simulink model "rl_17b"  (R2017b)
settings: Solver=VariableStepAuto  StartTime=0.0  StopTime=0.08  MaxStep=1e-4  RelTol=1e-8
values from neighbouring files (symbols this model uses):
  F_b = 50.0    (= 50)    [rl2_ini.m]    (also in rl_ini.m; rl_ini_jm.m; rlc_gformer_ini.m)
  L = 1e-3    (= 0.001)    [rl_ini.m]    (also in rl_ini_jm.m)
  Lmat = Lmat_km*Lenght    [rl_ini_jm.m]
  params_pu = [S_b,U_b,Omega_b,R,L]    [rl_ini.m]    (also in rl_ini_jm.m)
  R = 1.0    (= 1)    [rl_ini.m]    (also in rl_ini_jm.m)
  Rmat = Rmat_km*Lenght    [rl_ini_jm.m]
undefined symbols (not defined in the file or in its folder): T_s_power
libraries: powerlib x19, powerlib_meascontrol x8
settings Model: Creator=jmmauricio  LastModifiedBy=jmmau
settings CodeAppCC: StateflowObjectComments=on
settings SimscapeCC: SimscapeNormalizeSystem=off

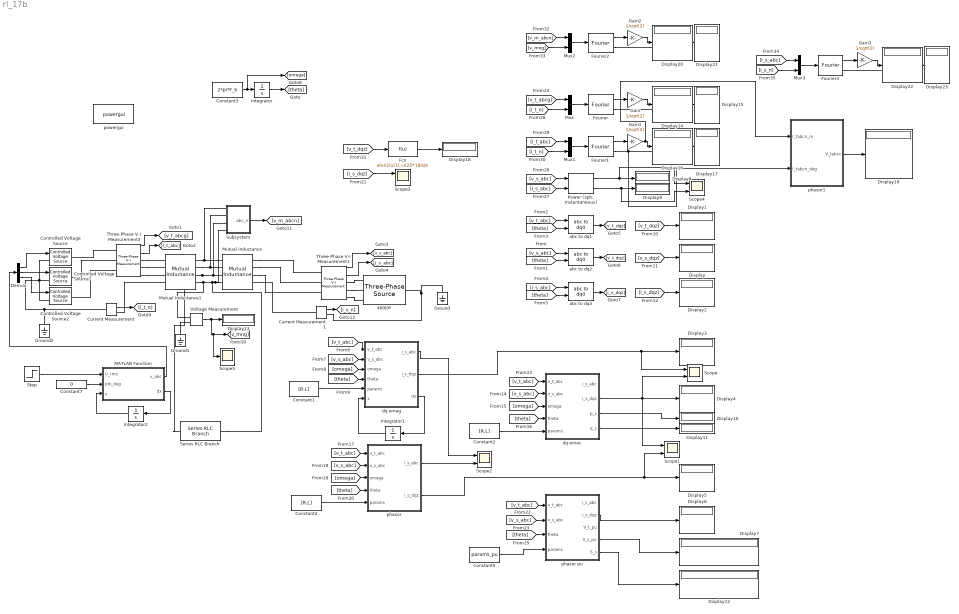
== system rl_17b ==
  400|0º : powerlib/Electrical Sources/Three-Phase Source  InternalConnection=Yn  VoltagePhases=off  Voltage=400  PhaseAngle=0  Voltage_phases=[25e3 25e3 25e3]/sqrt(3)  PhaseAngles_phases=[0 -120 +120]  Frequency=50  NonIdealSource=off  SpecifyImpedance=off  Resistance=0.8929  Inductance=16.58e-3  ShortCircuitLevel=100e6  BaseVoltage=25e3  XRratio=7  BusType=swing  Pref=10e3  Qref=0  Prefabc=[10e3, 10e3, 10e3]  Qrefabc=[0, 0, 0]  Qmin=-inf  Qmax=inf
  Constant1 : Constant  Value=[R,L]
  Constant2 : Constant  Value=[R,L]
  Constant3 : Constant  Value=2*pi*F_b
  Constant4 : Constant  Value=[R,L]
  Constant5 : Constant  Value=params_pu
  Constant7 : Constant  Value=0
  Controlled Voltage Source : powerlib/Electrical Sources/Controlled Voltage Source  Initialize=on  Source_Type=AC  Amplitude=0  Phase=0  Frequency=0  Measurements=None
  Controlled Voltage Source1 : powerlib/Electrical Sources/Controlled Voltage Source  Initialize=on  Source_Type=AC  Amplitude=0  Phase=0  Frequency=0  Measurements=None
  Controlled Voltage Source2 : powerlib/Electrical Sources/Controlled Voltage Source  Initialize=on  Source_Type=AC  Amplitude=0  Phase=0  Frequency=0  Measurements=None
  Current Measurement : powerlib/Measurements/Current Measurement  PhasorSimulation=off  OutputType=Complex  PSBequivalent=0
  Current Measurement1 : powerlib/Measurements/Current Measurement  PhasorSimulation=off  OutputType=Complex  PSBequivalent=0
  Demux : Demux  Outputs=3
  Display{,1..23} (24 alike) : Display
  Fcn : Fcn  Expr=atan2(u(1),-u(2))*180/pi
  Fourier{,1..3} (4 alike) : powerlib_meascontrol/Measurements/Fourier  Freq=50  n=1  InInit=[0, 0]  Ts=0
      settings: SourceProductName=Simscape Power Systems
  Gain{,1..3} (4 alike) : Gain  Gain=1/sqrt(2)
  Ground : powerlib/Elements/Ground  LConnTagsString=a
  Ground1 : powerlib/Elements/Ground  LConnTagsString=a
  Ground2 : powerlib/Elements/Ground  LConnTagsString=a
  Integrator : Integrator
  Integrator1 : Integrator  InitialCondition=[0,0]
  Integrator2 : Integrator  InitialCondition=0.0
  MATLAB Function : MATLAB Function  TreatAsAtomicUnit=on
  Mutual Inductance : powerlib/Elements/Mutual Inductance  LConnTagsString=a|b|c|L4  RConnTagsString=A|B|C|R4  TypeOfMutual=Generalized mutual inductance  NumberOfWindings=4  SelfImpedance1=[1.1 1.1e-03]  SelfImpedance2=[ 1.1 1.1e-03]  ThreeWindings=on  SelfImpedance3=[ 1.1 1.1e-03]  MutualImpedance=[1.0 1.0e-03]  InductanceMatrix=Lmat*35/315  ResistanceMatrix=Rmat*35/315  Measurements=None
      settings: AttributesFormatString=\n  SourceProductName=Simscape Power Systems  SourceProductBaseCode=PS
  Mutual Inductance1 : powerlib/Elements/Mutual Inductance  LConnTagsString=a|b|c|L4  RConnTagsString=A|B|C|R4  TypeOfMutual=Generalized mutual inductance  NumberOfWindings=4  SelfImpedance1=[1.1 1.1e-03]  SelfImpedance2=[ 1.1 1.1e-03]  ThreeWindings=on  SelfImpedance3=[ 1.1 1.1e-03]  MutualImpedance=[1.0 1.0e-03]  InductanceMatrix=Lmat*280/315  ResistanceMatrix=Rmat*280/315  Measurements=None
      settings: AttributesFormatString=\n  SourceProductName=Simscape Power Systems  SourceProductBaseCode=PS
  Mux{,1..3} (4 alike) : Mux  Inputs=2
  "Power (3ph, Instantaneous)" : powerlib_meascontrol/Measurements/Power (3ph, Instantaneous)
      settings: SourceProductName=Simscape Power Systems
  Scope{,1..4} (5 alike) : Scope  NumInputPorts=2
  Scope5 : Scope
  Series RLC Branch : powerlib/Elements/Series RLC Branch  LConnTagsString=__new0  RConnTagsString=__new0  BranchType=R  Resistance=2  Inductance=1e-3  SetiL0=off  InitialCurrent=0  Capacitance=1e-6  Setx0=off  InitialVoltage=0  Measurements=None
  Step : Step  Time=0.04  Before=400  After=400  SampleTime=0
  Subsystem : Subsystem
  Three-Phase V-I Measurement1 : powerlib/Measurements/Three-Phase V-I Measurement  VoltageMeasurement=phase-to-ground  SetLabelV=off  LabelV=Vabc  Vpu=off  VpuLL=off  CurrentMeasurement=yes  SetLabelI=off  LabelI=Iabc  Ipu=off  Pbase=100e6  Vbase=500e3  OutputType=Complex  PhasorSimulation=off  PSBequivalent=0
  Three-Phase V-I Measurement3 : powerlib/Measurements/Three-Phase V-I Measurement  VoltageMeasurement=phase-to-ground  SetLabelV=off  LabelV=Vabc  Vpu=off  VpuLL=off  CurrentMeasurement=yes  SetLabelI=off  LabelI=Iabc  Ipu=off  Pbase=100e6  Vbase=500e3  OutputType=Complex  PhasorSimulation=off  PSBequivalent=0
  Voltage Measurement : powerlib/Measurements/Voltage Measurement  PhasorSimulation=off  OutputType=Complex  PSBequivalent=0
  abc to dq1 : powerlib_meascontrol/Transformations/abc to dq0  Alignment=Aligned with phase A axis
  abc to dq2 : powerlib_meascontrol/Transformations/abc to dq0  Alignment=Aligned with phase A axis
  abc to dq3 : powerlib_meascontrol/Transformations/abc to dq0  Alignment=Aligned with phase A axis
  dq emag : MATLAB Function  TreatAsAtomicUnit=on
  dq emec : MATLAB Function  TreatAsAtomicUnit=on
  phasor : MATLAB Function  TreatAsAtomicUnit=on
  phasor pu : MATLAB Function  TreatAsAtomicUnit=on
  phasor1 : MATLAB Function  TreatAsAtomicUnit=on
  powergui : powerlib/powergui  Priority=1  SimulationMode=Continuous  SampleTime=T_s_power  frequency=60  Iterations=50  frequencyindice=50  Pbase=100e6  ErrMax=1e-4  UnitsV=kV  UnitsW=MW  buscounter=0  FunctionMessages=off  echomessages=off  EnableUseOfTLC=off  CurrentSourceSwitches=off  DisableSnubberDevices=off  DisableRonSwitches=off  DisableVfSwitches=off  DisplayEquations=off  SolverType=Tustin/Backward Euler (TBE)  Interpol=off  ExternalGateDelay=off  methode=off  Ts=100  x0status=blocks  SPID=on  SwTol=0  HookPort=off  RestoreLinks=warning  ResistiveCurrentMeasurement=off  Frange=[0:2:500]  Ylog=off  Xlog=on  ShowGrid=off  save=off  variable=ZData  structure=0  ZoomFFT=off  StartTime=0.0  cycles=1  DisplayStyle=1  fundamental=60  FreqAxis=off  MaxFrequency=1000  frequencyindicesteady=1  RmsSteady=1  display=off
  wires:
  Constant3/1 -> [omega], Integrator/1
  Integrator/1 -> [theta]
  Three-Phase V-I Measurement1/2 -> [i_s_abc]
  Three-Phase V-I Measurement1/1 -> [v_s_abc]
  [v_s_abc] -> abc to dq2/1
  [theta] -> abc to dq2/2
  [v_t_abc] -> abc to dq1/1
  [theta] -> abc to dq1/2
  [i_s_abc] -> abc to dq3/1
  [theta] -> abc to dq3/2
  abc to dq1/1 -> [v_t_dqz]
  abc to dq2/1 -> [v_s_dqz]
  abc to dq3/1 -> [i_s_dqz]
  [v_t_abc] -> dq emag/1(v_t_abc)
  [v_s_abc] -> dq emag/2(v_s_abc)
  [omega] -> dq emag/3(omega)
  [theta] -> dq emag/4(theta)
  Constant1/1 -> dq emag/5(params)
  Integrator1/1 -> dq emag/6(x)
  dq emag/3(dx) -> Integrator1/1
  [v_t_dqz] -> Display1/1
  [v_s_dqz] -> Display/1
  [i_s_dqz] -> Display2/1
  dq emag/2(i_s_dqz) -> Scope/1, Display3/1
  [v_s_abc] -> dq emec/2(v_s_abc)
  [omega] -> dq emec/3(omega)
  Constant2/1 -> dq emec/5(params)
  [v_t_abc] -> dq emec/1(v_t_abc)
  [theta] -> dq emec/4(theta)
  dq emec/2(i_s_dqz) -> Scope/2, Display4/1, Scope1/1
  [theta] -> phasor/4(theta)
  Constant4/1 -> phasor/5(params)
  [v_s_abc] -> phasor/2(v_s_abc)
  [omega] -> phasor/3(omega)
  [v_t_abc] -> phasor/1(v_t_abc)
  phasor/2(i_s_dqz) -> Scope1/2, Display5/1
  phasor/1(i_s_abc) -> Scope2/2
  dq emag/1(i_s_abc) -> Scope2/1
  [v_s_abc] -> phasor pu/2(v_s_abc)
  Constant5/1 -> phasor pu/4(params)
  [theta] -> phasor pu/3(theta)
  [v_t_abc] -> phasor pu/1(v_t_abc)
  phasor pu/2(i_s_dqz) -> Display6/1
  phasor pu/4(V_s_pu) -> Display7/1
  [v_s_abc] -> "Power (3ph, Instantaneous)"/1
  [i_s_abc] -> "Power (3ph, Instantaneous)"/2
  "Power (3ph, Instantaneous)"/2 -> Scope4/2, Display9/1
  "Power (3ph, Instantaneous)"/1 -> Scope4/1, Display8/1
  dq emec/4(q_s) -> Display11/1
  dq emec/3(p_s) -> Display10/1
  phasor pu/5(S_s) -> Display12/1
  Voltage Measurement/1 -> Scope5/1, [v_mng], Display13/1
  Demux/1 -> Controlled Voltage Source/1
  Demux/2 -> Controlled Voltage Source1/1
  Demux/3 -> Controlled Voltage Source2/1
  MATLAB Function/2(dx) -> Integrator2/1
  Integrator2/1 -> MATLAB Function/3(x)
  Step/1 -> MATLAB Function/1(U_rms)
  Constant7/1 -> MATLAB Function/2(phi_deg)
  MATLAB Function/1(v_abc) -> Demux/1
  Fourier/1 -> Gain/1
  Gain/1 -> Display14/1
  Fourier/2 -> Display15/1
  Current Measurement/1 -> [i_t_n]
  [v_t_abcg] -> Mux/1
  [i_t_n] -> Mux/2
  Mux/1 -> Fourier/1
  Mux1/1 -> Fourier1/1
  [i_t_n] -> Mux1/2
  [i_t_abc] -> Mux1/1
  Fourier1/2 -> Display17/1, phasor1/2(I_tabcn_deg)
  Gain1/1 -> phasor1/1(I_tabcn_m), Display16/1
  Fourier1/1 -> Gain1/1
  [v_t_dqz] -> Fcn/1
  Fcn/1 -> Display18/1
  [i_s_dqz] -> Scope3/1
  phasor1/1(V_tabcn) -> Display19/1
  Mux2/1 -> Fourier2/1
  [v_mng] -> Mux2/2
  [v_m_abcn] -> Mux2/1
  Fourier2/2 -> Display21/1
  Gain2/1 -> Display20/1
  Fourier2/1 -> Gain2/1
  Subsystem/1(abc_n) -> [v_m_abcn]
  Fourier3/1 -> Gain3/1
  Gain3/1 -> Display22/1
  Fourier3/2 -> Display23/1
  [i_s_abc] -> Mux3/1
  [i_s_n] -> Mux3/2
  Mux3/1 -> Fourier3/1
  Three-Phase V-I Measurement3/2 -> [i_t_abc]
  Three-Phase V-I Measurement3/1 -> [v_t_abcg]
  Current Measurement1/1 -> [i_s_n]
  connections:
  Three-Phase V-I Measurement1/RConn3 -- 400|0º/RConn3
  Three-Phase V-I Measurement1/RConn2 -- 400|0º/RConn2
  Three-Phase V-I Measurement1/RConn1 -- 400|0º/RConn1
  Ground1/LConn1 -- Voltage Measurement/LConn2
  Ground/LConn1 -- Current Measurement1/RConn1 -- 400|0º/LConn1
  Controlled Voltage Source2/LConn1 -- Current Measurement/LConn1 -- Ground2/LConn1 -- Controlled Voltage Source/LConn1 -- Controlled Voltage Source1/LConn1
  Mutual Inductance/RConn3 -- Three-Phase V-I Measurement1/LConn3
  Mutual Inductance/RConn2 -- Three-Phase V-I Measurement1/LConn2
  Mutual Inductance/RConn1 -- Three-Phase V-I Measurement1/LConn1
  Mutual Inductance1/RConn1 -- Subsystem/LConn1 -- Mutual Inductance/LConn1
  Mutual Inductance1/RConn2 -- Subsystem/LConn2 -- Mutual Inductance/LConn2
  Mutual Inductance1/RConn3 -- Series RLC Branch/LConn1 -- Subsystem/LConn3 -- Mutual Inductance/LConn3
  Mutual Inductance1/RConn4 -- Voltage Measurement/LConn1 -- Series RLC Branch/RConn1 -- Subsystem/LConn4 -- Mutual Inductance/LConn4
  Three-Phase V-I Measurement3/RConn1 -- Mutual Inductance1/LConn1
  Three-Phase V-I Measurement3/RConn2 -- Mutual Inductance1/LConn2
  Three-Phase V-I Measurement3/RConn3 -- Mutual Inductance1/LConn3
  Three-Phase V-I Measurement3/LConn3 -- Controlled Voltage Source2/RConn1
  Controlled Voltage Source1/RConn1 -- Three-Phase V-I Measurement3/LConn2
  Three-Phase V-I Measurement3/LConn1 -- Controlled Voltage Source/RConn1
  Mutual Inductance1/LConn4 -- Current Measurement/RConn1
  Current Measurement1/LConn1 -- Mutual Inductance/RConn4

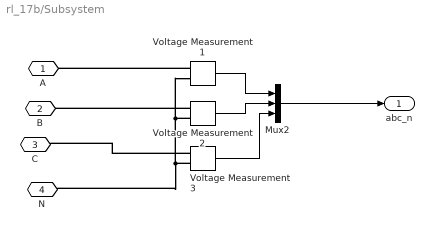
== system rl_17b/Subsystem ==
  Mux2 : Mux  Inputs=3
  Voltage Measurement1 : powerlib/Measurements/Voltage Measurement  PhasorSimulation=off  OutputType=Complex  PSBequivalent=0
  Voltage Measurement2 : powerlib/Measurements/Voltage Measurement  PhasorSimulation=off  OutputType=Complex  PSBequivalent=0
  Voltage Measurement3 : powerlib/Measurements/Voltage Measurement  PhasorSimulation=off  OutputType=Complex  PSBequivalent=0
  A : PMIOPort  Port=1  Side=Left
  B : PMIOPort  Port=2  Side=Left
  C : PMIOPort  Port=3  Side=Left
  N : PMIOPort  Port=4  Side=Left
  abc_n : Outport
  wires:
  Voltage Measurement3/1 -> Mux2/3
  Mux2/1 -> abc_n/1
  Voltage Measurement1/1 -> Mux2/1
  Voltage Measurement2/1 -> Mux2/2
  connections:
  Voltage Measurement2/LConn1 -- B/RConn1
  Voltage Measurement1/LConn1 -- A/RConn1
  Voltage Measurement3/LConn2 -- N/RConn1 -- Voltage Measurement2/LConn2 -- Voltage Measurement1/LConn2
  Voltage Measurement3/LConn1 -- C/RConn1

== matlab function rl_17b/dq emec ==
  data: v_t_abc input; i_s_abc output; i_s_dqz output; v_s_abc input; omega input; theta input; params input; p_s output; q_s output
function [i_s_abc,i_s_dqz,p_s,q_s] = fcn(v_t_abc,v_s_abc,omega,theta,params)

R = params(1);
L = params(2);

T_p = 2.0/3.0*[[ cos(theta), cos(theta-2.0/3.0*pi), cos(theta+2.0/3.0*pi)],
               [-sin(theta),-sin(theta-2.0/3.0*pi),-sin(theta+2.0/3.0*pi)],
               [        0.5,                   0.5,                   0.5]];
           

T_p_inv = [[            cos(theta),            -sin(theta), 1.0],
           [ cos(theta-2.0/3.0*pi), -sin(theta-2.0/3.0*pi), 1.0],
           [ cos(theta+2.0/3.0*pi), -sin(theta+2.0/3.0*pi), 1.0]];

v_t_dqz = T_p * v_t_abc;
v_s_dqz = T_p * v_s_abc;

v_t_d = v_t_dqz(1);
v_t_q = v_t_dqz(2);

v_s_d = v_s_dqz(1);
v_s_q = v_s_dqz(2);

i_s_d = -(R*v_s_d - R*v_t_d + L*omega*v_s_q - L*omega*v_t_q)/(L^2*omega^2 + R^2);
i_s_q = -(R*v_s_q - R*v_t_q - L*omega*v_s_d + L*omega*v_t_d)/(L^2*omega^2 + R^2);

i_s_dqz = [i_s_d,i_s_q,0].';

i_s_abc = T_p_inv * i_s_dqz;

p_s = 3/2*(i_s_d*v_s_d + i_s_q*v_s_q);
q_s = 3/2*(i_s_d*v_s_q - i_s_q*v_s_d);

== matlab function rl_17b/dq emag ==
  data: v_t_abc input; i_s_abc output; i_s_dqz output; v_s_abc input; omega input; theta input; params input; x input; dx output
function [i_s_abc,i_s_dqz,dx] = fcn(v_t_abc,v_s_abc,omega,theta,params,x)

R = params(1);
L = params(2);

T_p = 2.0/3.0*[[ cos(theta), cos(theta-2.0/3.0*pi), cos(theta+2.0/3.0*pi)],
               [-sin(theta),-sin(theta-2.0/3.0*pi),-sin(theta+2.0/3.0*pi)],
               [        0.5,                   0.5,                   0.5]];
           

T_p_inv = [[            cos(theta),            -sin(theta), 1.0],
           [ cos(theta-2.0/3.0*pi), -sin(theta-2.0/3.0*pi), 1.0],
           [ cos(theta+2.0/3.0*pi), -sin(theta+2.0/3.0*pi), 1.0]];

v_t_dqz = T_p * v_t_abc;
v_s_dqz = T_p * v_s_abc;

v_t_d = v_t_dqz(1);
v_t_q = v_t_dqz(2);

v_s_d = v_s_dqz(1);
v_s_q = v_s_dqz(2);

i_s_d = x(1);
i_s_q = x(2);

i_s_d = x(1);
i_s_q = x(2);

di_s_d = 1/L*(v_t_d - R*i_s_d + L*omega*i_s_q - v_s_d);
di_s_q = 1/L*(v_t_q - R*i_s_q - L*omega*i_s_d - v_s_q);

i_s_dqz = [i_s_d,i_s_q,0].';

i_s_abc = T_p_inv * i_s_dqz;

dx = [di_s_d; di_s_q];

== matlab function rl_17b/phasor ==
  data: v_t_abc input; i_s_abc output; i_s_dqz output; v_s_abc input; omega input; theta input; params input
function [i_s_abc,i_s_dqz] = fcn(v_t_abc,v_s_abc,omega,theta,params)

R = params(1);
L = params(2);

T_p = 2.0/3.0*[[ cos(theta), cos(theta-2.0/3.0*pi), cos(theta+2.0/3.0*pi)],
               [-sin(theta),-sin(theta-2.0/3.0*pi),-sin(theta+2.0/3.0*pi)],
               [        0.5,                   0.5,                   0.5]];
           

T_p_inv = [[            cos(theta),            -sin(theta), 1.0],
           [ cos(theta-2.0/3.0*pi), -sin(theta-2.0/3.0*pi), 1.0],
           [ cos(theta+2.0/3.0*pi), -sin(theta+2.0/3.0*pi), 1.0]];

v_t_dqz = T_p * v_t_abc;
v_s_dqz = T_p * v_s_abc;

v_t_i =  v_t_dqz(1)/sqrt(2);
v_t_r = -v_t_dqz(2)/sqrt(2);

V_t = v_t_r + 1i*v_t_i;

v_s_i =  v_s_dqz(1)/sqrt(2);
v_s_r = -v_s_dqz(2)/sqrt(2);

V_s = v_s_r + 1i*v_s_i;

X = L*omega;
Z = R + 1j*X;

I_s = (V_t - V_s)/Z;

i_s_d = sqrt(2)*imag(I_s);
i_s_q =-sqrt(2)*real(I_s);

i_s_dqz = [i_s_d,i_s_q,0].';

i_s_abc = T_p_inv * i_s_dqz;

== matlab function rl_17b/phasor pu ==
  data: v_t_abc input; i_s_abc output; i_s_dqz output; v_s_abc input; theta input; params input; V_t_pu output; V_s_pu output; S_s output
function [i_s_abc,i_s_dqz,V_t_pu,V_s_pu,S_s] = fcn(v_t_abc,v_s_abc,theta,params)

S_b = params(1);
U_b = params(2);
Omega_b = params(3);
R = params(4);
L = params(5);


V_b_dq = U_b*sqrt(2/3);
I_b_dq = S_b/U_b*sqrt(2/3);
Z_b = U_b^2/S_b;

R_pu = R/Z_b;
X_pu = Omega_b*L/Z_b;


T_p = 2.0/3.0*[[ cos(theta), cos(theta-2.0/3.0*pi), cos(theta+2.0/3.0*pi)],
               [-sin(theta),-sin(theta-2.0/3.0*pi),-sin(theta+2.0/3.0*pi)],
               [        0.5,                   0.5,                   0.5]];
           

T_p_inv = [[            cos(theta),            -sin(theta), 1.0],
           [ cos(theta-2.0/3.0*pi), -sin(theta-2.0/3.0*pi), 1.0],
           [ cos(theta+2.0/3.0*pi), -sin(theta+2.0/3.0*pi), 1.0]];

v_t_dqz = T_p * v_t_abc;
v_s_dqz = T_p * v_s_abc;

v_t_i_pu =  v_t_dqz(1)/V_b_dq;
v_t_r_pu = -v_t_dqz(2)/V_b_dq;

V_t_pu = v_t_r_pu + 1i*v_t_i_pu;

v_s_i_pu =  v_s_dqz(1)/V_b_dq;
v_s_r_pu = -v_s_dqz(2)/V_b_dq;

V_s_pu = v_s_r_pu + 1i*v_s_i_pu;


Z_pu = R_pu + 1j*X_pu;

I_s_pu = (V_t_pu - V_s_pu)/Z_pu;

i_s_d = I_b_dq*imag(I_s_pu);
i_s_q =-I_b_dq*real(I_s_pu);

i_s_dqz = [i_s_d,i_s_q,0].';

i_s_abc = T_p_inv * i_s_dqz;

S_s_pu = V_s_pu*conj(I_s_pu);
S_s = S_s_pu*S_b;

== matlab function rl_17b/MATLAB Function ==
  data: U_rms input; v_abc output; phi_deg input; x input; dx output
function [v_abc,dx] = fcn(U_rms,phi_deg,x)

%theta=0;
theta = x;
theta_e = theta + phi_deg*pi/180;
v_amp = U_rms*sqrt(2/3);
v_abc = v_amp*[sin(theta_e);sin(theta_e-2/3*pi);sin(theta_e-4/3*pi)];
%v_abc = [0,0,0].';
dx = 2*pi*50.0;

== matlab function rl_17b/phasor1 ==
  data: I_tabcn_m input; V_tabcn output; I_tabcn_deg input
function V_tabcn  = fcn(I_tabcn_m,I_tabcn_deg)

I_tabcn_rad = I_tabcn_deg/180*pi;
I_tabcn = I_tabcn_m.*(cos(I_tabcn_rad) + 1j*sin(I_tabcn_rad));
Omega_b = 2*pi*50.0;
Lenght = 0.315
% CIGRE UG1
Rmat_km = [[ 0.211,  0.049,  0.049,  0.049],
        [ 0.049,  0.211,  0.049,  0.049],
        [ 0.049,  0.049,  0.211,  0.049],
        [ 0.049,  0.049,  0.049,  0.211]];
Xmat_km =[[ 0.747,  0.673,  0.651,  0.673],
       [ 0.673,  0.747,  0.673,  0.651],
       [ 0.651,  0.673,  0.747,  0.673],
       [ 0.673,  0.651,  0.673,  0.747]];
   

Lmat_km = Xmat_km/Omega_b;

Rmat = Rmat_km*Lenght;
Xmat = Lmat_km*Omega_b*Lenght;

Zmat = Rmat + 1j* Xmat;

sinus =  [(cos(0       ) + 1j*sin(0       )),
          (cos(0-2/3*pi) + 1j*sin(0-2/3*pi)),
          (cos(0+2/3*pi) + 1j*sin(0+2/3*pi))
          0.0].';
V_tabcn = abs(Zmat*I_tabcn + 400.0/sqrt(3)*sinus.');
